simulink model "voter"  (R2024b)
settings: Solver=FixedStepAuto  StartTime=0.0  StopTime=20  RelTol=1e-3
settings Model: Creator=aayan  LastModifiedBy=aayan
settings ConfigComp: CovEnable=on  RecordCoverage=on  CovMetricSettings=dcmwe  CovModelRefEnable=on

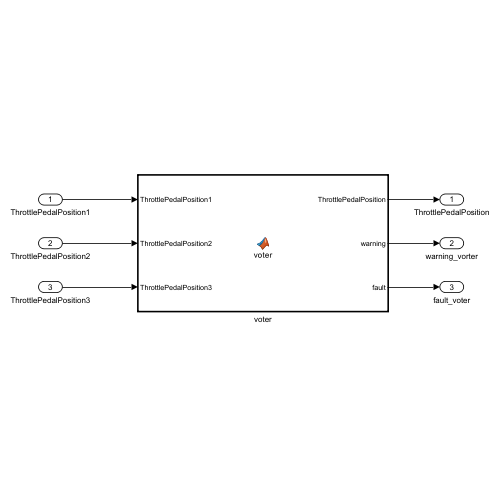
[thumbnail: Simulink's stored preview of the top-level diagram]
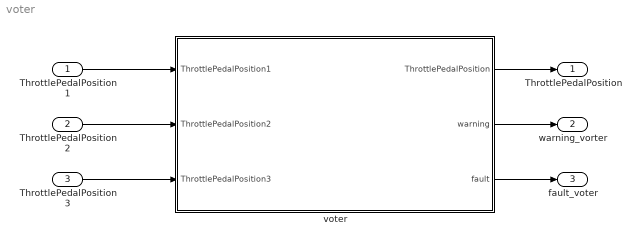
== system voter ==
  ThrottlePedalPosition1 : Inport  OutDataTypeStr=single
  ThrottlePedalPosition2 : Inport  Port=2  OutDataTypeStr=single
  ThrottlePedalPosition3 : Inport  Port=3  OutDataTypeStr=single
  voter : MATLAB Function  TreatAsAtomicUnit=on
  ThrottlePedalPosition : Outport
  warning_vorter : Outport  Port=2  OutDataTypeStr=boolean
  fault_voter : Outport  Port=3  OutDataTypeStr=boolean
  wires:
  voter/2(warning) -> warning_vorter/1
  voter/3(fault) -> fault_voter/1
  ThrottlePedalPosition1/1 -> voter/1(ThrottlePedalPosition1)
  ThrottlePedalPosition2/1 -> voter/2(ThrottlePedalPosition2)
  ThrottlePedalPosition3/1 -> voter/3(ThrottlePedalPosition3)
  voter/1(ThrottlePedalPosition) -> ThrottlePedalPosition/1

== matlab function voter/voter ==
  data: ThrottlePedalPosition output; ThrottlePedalPosition1 input; warning output; fault output; ThrottlePedalPosition2 input; ThrottlePedalPosition3 input
function [ThrottlePedalPosition,warning, fault] = voter( ...
    ThrottlePedalPosition1,ThrottlePedalPosition2,ThrottlePedalPosition3)
% initialization
warning = boolean(0);
fault = boolean(0);
ThrottlePedalPosition = single(0);

if (abs(ThrottlePedalPosition1 - ThrottlePedalPosition2) > 0.025)
    % one sensor might be faulty

    if(abs(ThrottlePedalPosition1 - ThrottlePedalPosition3) > 0.025)
        if(abs(ThrottlePedalPosition2 - ThrottlePedalPosition3) > 0.025)
            % all three differ
            warning = boolean(1);
            fault = boolean(1); 
            ThrottlePedalPosition = single(0);
        else
            % sensor 1 is faulty
            warning = boolean(1);
            ThrottlePedalPosition = mean([ThrottlePedalPosition2,ThrottlePedalPosition3]);
        end
    else %1 and 3 consistent
        if(abs(ThrottlePedalPosition2 - ThrottlePedalPosition3) > 0.025)
            % sensor 2 is faulty
            warning = boolean(1);
            ThrottlePedalPosition = mean([ThrottlePedalPosition1,ThrottlePedalPosition3]);
        else
            % 3 in the middle
            warning = boolean(1);
            ThrottlePedalPosition = mean([ThrottlePedalPosition1,ThrottlePedalPosition2,ThrottlePedalPosition3]);
        end
    end
    
else
    % sensors 1 and 2 are within range
    if(abs(ThrottlePedalPosition1 - ThrottlePedalPosition3) > 0.025)
        if(abs(ThrottlePedalPosition2 - ThrottlePedalPosition3) > 0.025)
            % sensor 3 is faulty
            warning = boolean(1);
            ThrottlePedalPosition = mean([ThrottlePedalPosition1,ThrottlePedalPosition2]);
        else
            % 2 in the middle
            ThrottlePedalPosition = mean([ThrottlePedalPosition1,ThrottlePedalPosition2,ThrottlePedalPosition3]);

        end
    else
        % all sensors are close enough
        ThrottlePedalPosition = mean([ThrottlePedalPosition1,ThrottlePedalPosition2,ThrottlePedalPosition3]);
    end
end
